simulink model "SchemaIntegrateurQ3a"  (R2025b)
settings: Solver=VariableStepAuto  StartTime=0.0  StopTime=35  RelTol=1e-3
undefined symbols (not defined in the file or in its folder): g0, he, Kd, Kf, Kp, L, m, R, ue
settings Model: Creator=Louis  LastModifiedBy=Louis

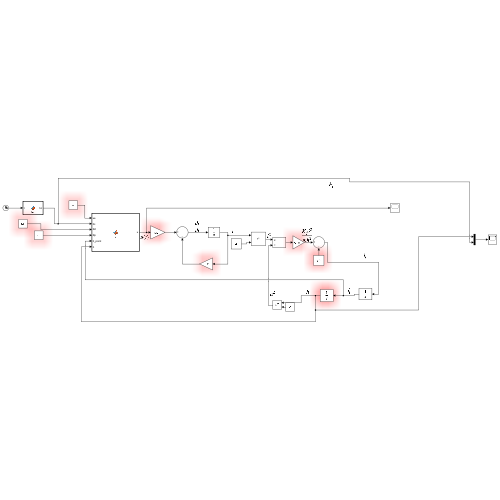
[thumbnail: Simulink's stored preview of the top-level diagram]
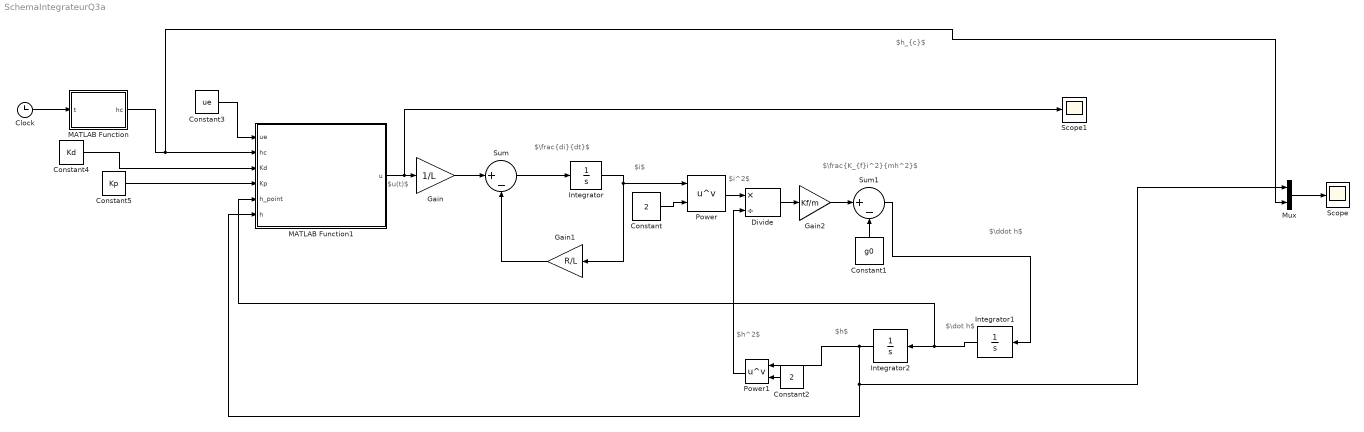
== system SchemaIntegrateurQ3a ==
  note: $h_{c}$
  note: $h^2$
  note: $h$
  note: $\dot h$
  note: $\ddot h$
  note: $\frac{K_{f}i^2}{mh^2}$
  note: $i^2$
  note: $i$
  note: $\frac{di}{dt}$
  note: $u(t)$
  Clock : Clock
  Constant : Constant  Value=2
  Constant1 : Constant  Value=g0
  Constant2 : Constant  Value=2
  Constant3 : Constant  Value=ue
  Constant4 : Constant  Value=Kd
  Constant5 : Constant  Value=Kp
  Divide : Product  Inputs=*/
  Gain : Gain  Gain=1/L
  Gain1 : Gain  Gain=R/L
  Gain2 : Gain  Gain=Kf/m
  Integrator : Integrator  InitialCondition=1.5
  Integrator1 : Integrator
  Integrator2 : Integrator  InitialCondition=he
  MATLAB Function : MATLAB Function  TreatAsAtomicUnit=on
  MATLAB Function1 : MATLAB Function  TreatAsAtomicUnit=on
  Mux : Mux  Inputs=2
  Power : Math  Operator=pow
  Power1 : Math  Operator=pow
  Scope : Scope
      settings: ActiveDisplayYMinimum=-66228.785032176937  ActiveDisplayYMaximum=596055.23456332588  DataLoggingVariableName=h_hc_t  DataLoggingSaveFormat=Array
  Scope1 : Scope
      settings: ActiveDisplayYMinimum=-1  ActiveDisplayYMaximum=1  DataLoggingVariableName=u_t  DataLoggingSaveFormat=Array
  Sum : Sum  Inputs=|+-
  Sum1 : Sum  Inputs=|+-
  wires:
  Gain/1 -> Sum/1
  Gain1/1 -> Sum/2
  Sum/1 -> Integrator/1
  Integrator/1 -> Power/1, Gain1/1
  Constant/1 -> Power/2
  Power/1 -> Divide/1
  Divide/1 -> Gain2/1
  Constant1/1 -> Sum1/2
  Mux/1 -> Scope/1
  Sum1/1 -> Integrator1/1
  Integrator1/1 -> MATLAB Function1/5(h_point), Integrator2/1
  Integrator2/1 -> Mux/1, MATLAB Function1/6(h), Power1/1
  Constant2/1 -> Power1/2
  Power1/1 -> Divide/2
  Gain2/1 -> Sum1/1
  Clock/1 -> MATLAB Function/1(t)
  MATLAB Function/1(hc) -> MATLAB Function1/2(hc), Mux/2
  MATLAB Function1/1(u) -> Scope1/1, Gain/1
  Constant3/1 -> MATLAB Function1/1(ue)
  Constant5/1 -> MATLAB Function1/4(Kp)
  Constant4/1 -> MATLAB Function1/3(Kd)

== matlab function SchemaIntegrateurQ3a/MATLAB Function1 ==
  data: ue input; hc input; Kd input; Kp input; u output; h_point input; h input
function u = u( ue, hc, Kd, Kp,h_point,h)
u = ue - Kd*h_point -Kp*(h - hc);
end

== matlab function SchemaIntegrateurQ3a/MATLAB Function ==
  data: t input; hc output
function hc = hc(t)
    
if (0 <= t) && (t < 5) 
    hc = -0.05;
elseif (5 <= t) && (t < 10)
    hc = -0.075;
elseif (10 <= t) && (t < 15)
    hc = -0.06;
elseif (15 <= t) && (t < 20)
    hc = -0.055;
else
    hc = -0.05;
end
